simulink model "ship_p5"  (R2014a)
settings: Solver=ode45  StartTime=0.0  StopTime=500  RelTol=1e-3
undefined symbols (not defined in the file): Ad, alpha, Bd, C, K_pd, P0_apriori, Q_wd, R_v, T, T_sam, x0_apriori
libraries: dspinverses x4, dspmtrx3 x2, dspsrcs4 x2, simulink x1
settings Model: CovSFcnEnable=on  Creator=markh  LastModifiedBy=alexada
settings DataIOCC: SignalLoggingSaveFormat=ModelDataLogs  SignalLoggingName=sigsOut
settings OptimizationCC: InitFltsAndDblsToZero=on
settings DebuggingCC: SaveWithParameterizedLinksMsg=none  UnderspecifiedInitializationDetection=Classic  SignalResolutionControl=TryResolveAllWithWarning  SolverPrmCheckMsg=none  MultiTaskDSMMsg=warning  MultiTaskCondExecSysMsg=none  FcnCallInpInsideContextMsg=UseLocalSettings  FrameProcessingCompatibilityMsg=error  StateNameClashWarn=warning
settings HardwareCC: TargetUnknown=on
settings GRTTargetCC: TargetFcnLib=ansi_tfl_tmw.mat  CombineOutputUpdateFcns=off  GRTInterface=on

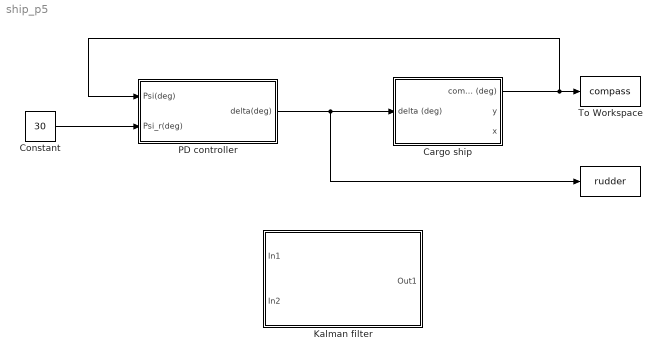
== system ship_p5 ==
  " " : ToWorkspace  VariableName=rudder  SaveFormat=Timeseries  SampleTime=-1
  Cargo ship : Subsystem  mask(Simple shipmodel for a cargo ship){noise=on, current=on, waves=off}
      mask prompts: noise "measurement noise"
      mask help:
      | Measurement noise:
      | 	checked = noise on
      | 	unchecked = noise off
      |
      | Current:
      | 	checked = current on
      | 	unchecked = current off
      |
      | Waves:
      | 	checked = waves on
      | 	unchecked = waves off
      |
      | Author: Jørgen Spjøtvold, 9/10-2003
      | TTK 4115 Linear system theory.
      | Modified by Jostein Bakkeheim 26/10-2006
  Constant : Constant  Value=30
  Kalman filter : Subsystem
  PD controller : Subsystem
  To Workspace : ToWorkspace  VariableName=compass  SaveFormat=Timeseries  SampleTime=-1
  wires:
  Cargo ship/1(compass (deg)) -> PD controller/1(Psi(deg)), To Workspace/1
  Constant/1 -> PD controller/2(Psi_r(deg))
  PD controller/1(delta(deg)) -> Cargo ship/1(delta (deg)), " "/1

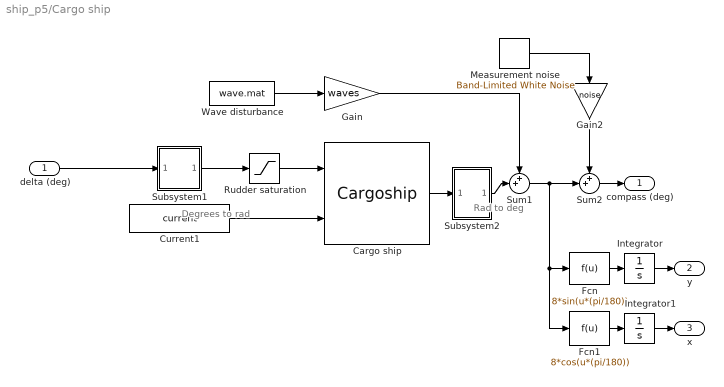
== system ship_p5/Cargo ship ==
  note: Degrees to rad
  note: Rad to deg
  delta (deg) : Inport
  Cargo ship : S-Function  FunctionName=Cargoship  EnableBusSupport=off  mask(Cargo ship){}
      mask help:
      | S-function which simulates a cargo ship.
      |
      | Author: Jørgen Spjøtvold
      | 20.10-2003
      | Modified by Jostein Bakkeheim 27.10.2006
  Current1 : Constant  Value=current
  Fcn : Fcn  Expr=8*sin(u*(pi/180))
  Fcn1 : Fcn  Expr=8*cos(u*(pi/180))
  Gain : Gain  Gain=waves  SaturateOnIntegerOverflow=on  OutDataTypeStr=Inherit: Same as input  ParamDataTypeStr=Inherit: Same as input
  Gain2 : Gain  Gain=noise  SaturateOnIntegerOverflow=on  OutDataTypeStr=Inherit: Same as input  ParamDataTypeStr=Inherit: Same as input
  Integrator : Integrator
  Integrator1 : Integrator
  Measurement noise : simulink/Sources/Band-Limited White Noise  Cov=[0.001]  Ts=.5  seed=[23341]
  Rudder saturation : Saturate  UpperLimit=45*(pi/180)  LowerLimit=-45*(pi/180)
  Subsystem1 : Subsystem  mask(degrees to radians){}
      mask help: Converts degrees to radians
      mask Display: fprintf('D2R');
  Subsystem2 : Subsystem  mask(radians to degrees){}
      mask help: Converts radians to degrees
      mask Display: fprintf('R2D');
  Sum1 : Sum  Inputs=++|  SaturateOnIntegerOverflow=on
  Sum2 : Sum  Inputs=++|  SaturateOnIntegerOverflow=on
  Wave disturbance : FromFile  FileName=wave.mat  SampleTime=0
  compass (deg) : Outport
  y : Outport  Port=2
  x : Outport  Port=3
  wires:
  delta (deg)/1 -> Subsystem1/1(In1)
  Fcn/1 -> Integrator/1
  Integrator/1 -> y/1
  Fcn1/1 -> Integrator1/1
  Integrator1/1 -> x/1
  Wave disturbance/1 -> Gain/1
  Subsystem2/1(Out1) -> Sum1/2
  Gain/1 -> Sum1/1
  Sum1/1 -> Fcn/1, Fcn1/1, Sum2/2
  Cargo ship/1 -> Subsystem2/1(In1)
  Subsystem1/1(Out1) -> Rudder saturation/1
  Rudder saturation/1 -> Cargo ship/1
  Sum2/1 -> compass (deg)/1
  Measurement noise/1 -> Gain2/1
  Gain2/1 -> Sum2/1
  Current1/1 -> Cargo ship/2

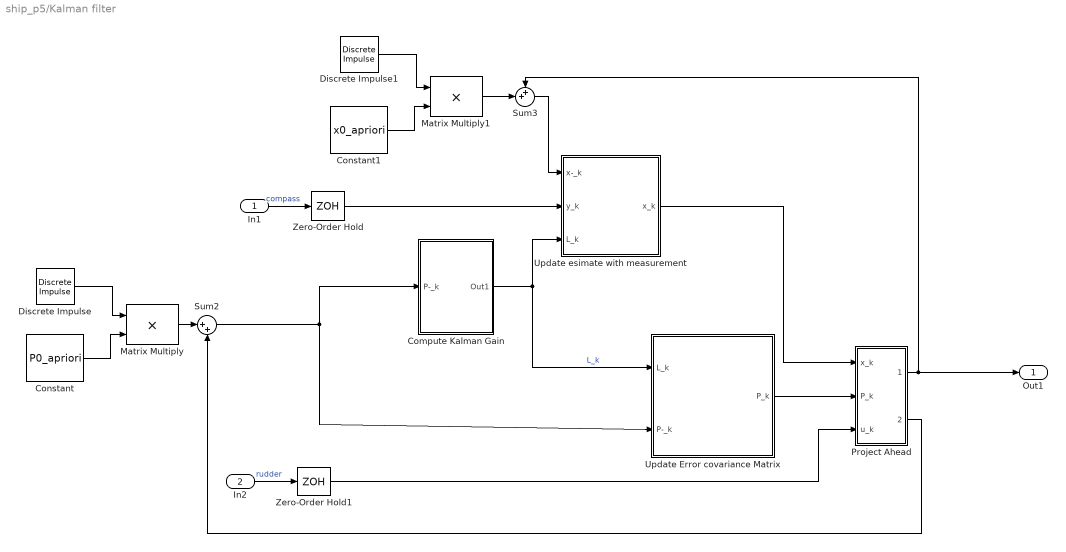
== system ship_p5/Kalman filter ==
  In1 : Inport
  In2 : Inport  Port=2
  Compute Kalman Gain : Subsystem
  Constant : Constant  Value=P0_apriori  VectorParams1D=off
  Constant1 : Constant  Value=x0_apriori  VectorParams1D=off
  Discrete Impulse : dspsrcs4/Discrete  Impulse  Delay=0  SampleTime=1  FrameSample=1  dataType=double  isSigned=on  wordLen=16  udDataType=sfix(16)  fracBitsMode=Best precision  numFracBits=15  OutDataTypeStr=double  LastOutDataTypeStr=double
  Discrete Impulse1 : dspsrcs4/Discrete  Impulse  Delay=0  SampleTime=1  FrameSample=1  dataType=double  isSigned=on  wordLen=16  udDataType=sfix(16)  fracBitsMode=Best precision  numFracBits=15  OutDataTypeStr=double  LastOutDataTypeStr=double
  Matrix Multiply : Product
  Matrix Multiply1 : Product
  Project Ahead : Subsystem
  Sum2 : Sum  Inputs=|++
  Sum3 : Sum  Inputs=++|
  Update Error covariance Matrix : Subsystem
  Update esimate with measurement : Subsystem
  Zero-Order Hold : ZeroOrderHold  SampleTime=T_sam
  Zero-Order Hold1 : ZeroOrderHold  SampleTime=T_sam
  Out1 : Outport
  wires:
  In1/1 -> Zero-Order Hold/1  "compass"
  In2/1 -> Zero-Order Hold1/1  "rudder"
  Zero-Order Hold/1 -> Update esimate with measurement/2(y_k)
  Compute Kalman Gain/1(Out1) -> Update Error covariance Matrix/1(L_k), Update esimate with measurement/3(L_k)  "L_k"
  Discrete Impulse/1 -> Matrix Multiply/1
  Constant/1 -> Matrix Multiply/2
  Matrix Multiply/1 -> Sum2/1
  Discrete Impulse1/1 -> Matrix Multiply1/1
  Constant1/1 -> Matrix Multiply1/2
  Update esimate with measurement/1(x_k) -> Project Ahead/1(x_k)
  Update Error covariance Matrix/1(P_k) -> Project Ahead/2(P_k)
  Zero-Order Hold1/1 -> Project Ahead/3(u_k)
  Project Ahead/1(x-_k+1) -> Sum3/1, Out1/1
  Project Ahead/2(P-_k+1) -> Sum2/2
  Sum2/1 -> Update Error covariance Matrix/2(P-_k), Compute Kalman Gain/1(P-_k)
  Sum3/1 -> Update esimate with measurement/1(x-_k)
  Matrix Multiply1/1 -> Sum3/2

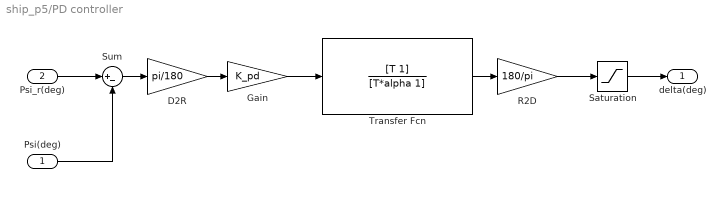
== system ship_p5/PD controller ==
  Psi(deg) : Inport
  Psi_r(deg) : Inport  Port=2
  D2R : Gain  Gain=pi/180
  Gain : Gain  Gain=K_pd
  R2D : Gain  Gain=180/pi
  Saturation : Saturate  UpperLimit=45  LowerLimit=-45
  Sum : Sum  Inputs=|+-
  Transfer Fcn : TransferFcn  Numerator=[T 1]  Denominator=[T*alpha 1]
  delta(deg) : Outport
  wires:
  Psi_r(deg)/1 -> Sum/1
  Psi(deg)/1 -> Sum/2
  Gain/1 -> Transfer Fcn/1
  Sum/1 -> D2R/1
  D2R/1 -> Gain/1
  Transfer Fcn/1 -> R2D/1
  R2D/1 -> Saturation/1
  Saturation/1 -> delta(deg)/1

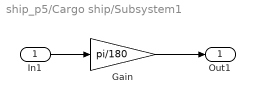
== system ship_p5/Cargo ship/Subsystem1 ==
  In1 : Inport
  Gain : Gain  Gain=pi/180  SaturateOnIntegerOverflow=on  OutDataTypeStr=Inherit: Same as input  ParamDataTypeStr=Inherit: Same as input
  Out1 : Outport
  wires:
  Gain/1 -> Out1/1
  In1/1 -> Gain/1

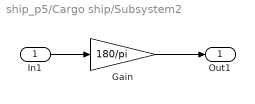
== system ship_p5/Cargo ship/Subsystem2 ==
  In1 : Inport
  Gain : Gain  Gain=180/pi  SaturateOnIntegerOverflow=on  OutDataTypeStr=Inherit: Same as input  ParamDataTypeStr=Inherit: Same as input
  Out1 : Outport
  wires:
  Gain/1 -> Out1/1
  In1/1 -> Gain/1

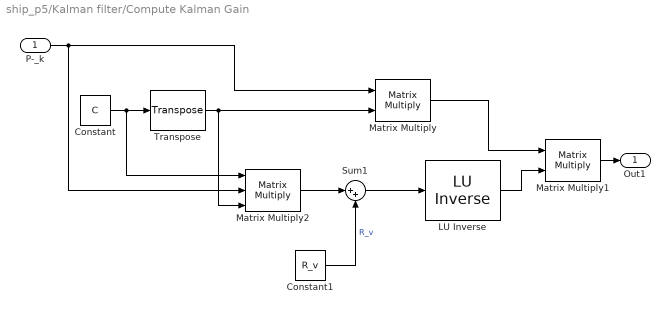
== system ship_p5/Kalman filter/Compute Kalman Gain ==
  P-_k : Inport
  " LU Inverse" : dspinverses/ LU Inverse
  Constant : Constant  Value=C  VectorParams1D=off
  Constant1 : Constant  Value=R_v  VectorParams1D=off
  Matrix Multiply : Product  Multiplication=Matrix(*)
  Matrix Multiply1 : Product  Multiplication=Matrix(*)
  Matrix Multiply2 : Product  Inputs=3  Multiplication=Matrix(*)
  Sum1 : Sum  Inputs=|++
  Transpose : dspmtrx3/Transpose  Hermitian=off  overflowFlag=off
  Out1 : Outport
  wires:
  Transpose/1 -> Matrix Multiply2/3, Matrix Multiply/2
  Matrix Multiply/1 -> Matrix Multiply1/1
  Constant1/1 -> Sum1/2  "R_v"
  Sum1/1 -> " LU Inverse"/1
  Matrix Multiply1/1 -> Out1/1
  P-_k/1 -> Matrix Multiply2/2, Matrix Multiply/1
  " LU Inverse"/1 -> Matrix Multiply1/2
  Matrix Multiply2/1 -> Sum1/1
  Constant/1 -> Matrix Multiply2/1, Transpose/1

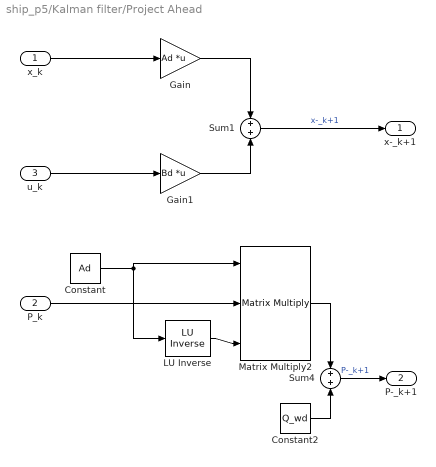
== system ship_p5/Kalman filter/Project Ahead ==
  x_k : Inport
  P_k : Inport  Port=2
  u_k : Inport  Port=3
  " LU Inverse" : dspinverses/ LU Inverse
  Constant : Constant  Value=Ad  VectorParams1D=off
  Constant2 : Constant  Value=Q_wd  VectorParams1D=off
  Gain : Gain  Gain=Ad  Multiplication=Matrix(K*u)
  Gain1 : Gain  Gain=Bd  Multiplication=Matrix(K*u)
  Matrix Multiply2 : Product  Inputs=3  Multiplication=Matrix(*)
  Sum1 : Sum  Inputs=+|+
  Sum4 : Sum  Inputs=+|+
  x-_k+1 : Outport
  P-_k+1 : Outport  Port=2
  wires:
  Sum4/1 -> P-_k+1/1  "P-_k+1"
  Constant2/1 -> Sum4/2
  u_k/1 -> Gain1/1
  x_k/1 -> Gain/1
  Gain1/1 -> Sum1/2
  Gain/1 -> Sum1/1
  Sum1/1 -> x-_k+1/1  "x-_k+1"
  P_k/1 -> Matrix Multiply2/2
  Matrix Multiply2/1 -> Sum4/1
  " LU Inverse"/1 -> Matrix Multiply2/3
  Constant/1 -> " LU Inverse"/1, Matrix Multiply2/1

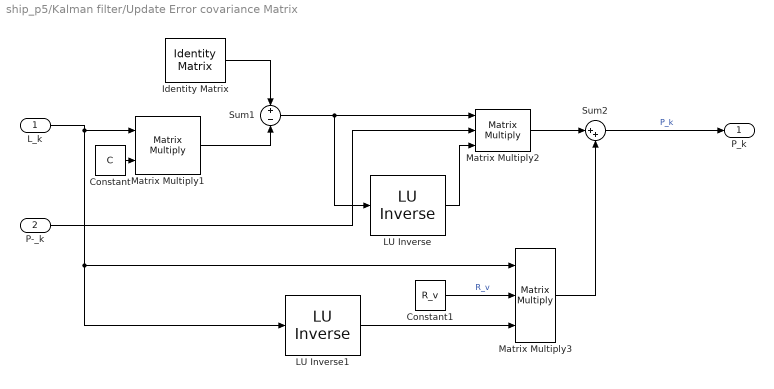
== system ship_p5/Kalman filter/Update Error covariance Matrix ==
  L_k : Inport
  P-_k : Inport  Port=2
  " LU Inverse" : dspinverses/ LU Inverse
  " LU Inverse1" : dspinverses/ LU Inverse
  Constant : Constant  Value=C  VectorParams1D=off
  Constant1 : Constant  Value=R_v  VectorParams1D=off
  Identity Matrix : dspmtrx3/Identity Matrix  Inherit=off  N=5  Ts=1  dataType=double  isSigned=on  wordLen=16  udDataType=sfix(16)  fracBitsMode=Best precision  numFracBits=15  OutDataTypeStr=double  LastOutDataTypeStr=double
  Matrix Multiply1 : Product  Multiplication=Matrix(*)
  Matrix Multiply2 : Product  Inputs=3  Multiplication=Matrix(*)
  Matrix Multiply3 : Product  Inputs=3  Multiplication=Matrix(*)
  Sum1 : Sum  Inputs=+|-
  Sum2 : Sum  Inputs=|++
  P_k : Outport
  wires:
  Constant/1 -> Matrix Multiply1/2
  Identity Matrix/1 -> Sum1/1
  Constant1/1 -> Matrix Multiply3/2  "R_v"
  Sum1/1 -> " LU Inverse"/1, Matrix Multiply2/1
  L_k/1 -> Matrix Multiply1/1, Matrix Multiply3/1, " LU Inverse1"/1
  Matrix Multiply1/1 -> Sum1/2
  Sum2/1 -> P_k/1  "P_k"
  P-_k/1 -> Matrix Multiply2/2
  " LU Inverse"/1 -> Matrix Multiply2/3
  Matrix Multiply2/1 -> Sum2/1
  " LU Inverse1"/1 -> Matrix Multiply3/3
  Matrix Multiply3/1 -> Sum2/2

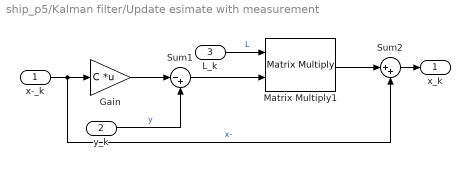
== system ship_p5/Kalman filter/Update esimate with measurement ==
  x-_k : Inport
  y_k : Inport  Port=2
  L_k : Inport  Port=3
  Gain : Gain  Gain=C  Multiplication=Matrix(K*u)
  Matrix Multiply1 : Product  Multiplication=Matrix(*)
  Sum1 : Sum  Inputs=|-+
  Sum2 : Sum  Inputs=|++
  x_k : Outport
  wires:
  x-_k/1 -> Sum2/2, Gain/1  "x-"
  y_k/1 -> Sum1/2  "y"
  Sum1/1 -> Matrix Multiply1/2
  Sum2/1 -> x_k/1
  Matrix Multiply1/1 -> Sum2/1
  Gain/1 -> Sum1/1
  L_k/1 -> Matrix Multiply1/1  "L"
